simulink library "NonEntVncAppliedBtc"  (R2022b)
settings: Solver=VariableStepAuto  StartTime=0.0  StopTime=10.0  RelTol=1e-3
values from neighbouring files (symbols this model uses):
  den = [b1 b2]    [firstOrderButter.m]
  num = [a1 a2]    [firstOrderButter.m]
undefined symbols (not defined in the file or in its folder): Row
libraries: TuneVar x4, TOP x2, FeaturePath x1, HandyTextFile x1, dspsigops x1, AudioStats x1
settings Model: Creator=kl13806  LastModifiedBy=kl13806
settings SolverCC: AlgebraicLoopSolver=TrustRegion
settings DebuggingCC: UnconnectedInputMsg=warning  UnconnectedOutputMsg=warning  UnconnectedLineMsg=warning  SFMachineParentedDataDiag=warning
settings ModelReferenceCC: EnableRefExpFcnMdlSchedulingChecks=on
settings RTWCC: DLArmComputeVersion=19.05

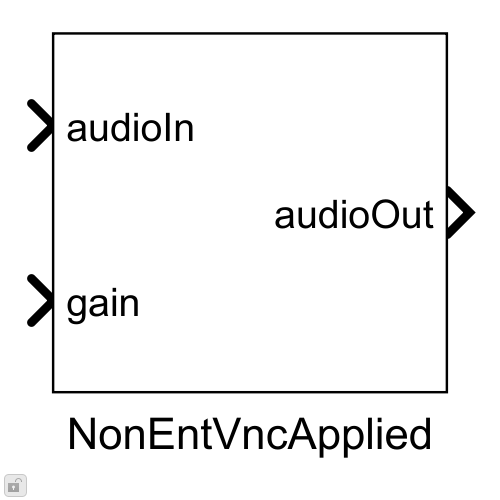
[thumbnail: Simulink's stored preview of the top-level diagram]
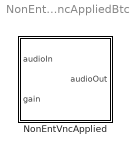
== system NonEntVncAppliedBtc ==
  NonEntVncApplied : Subsystem  mask(Blocklib NonEntVncApplied){Config=[], FeatureName=VNC}
      mask prompts: Config "NonEntVncAppliedConfig"; FeatureName "Feature path name:"
      mask init:
      | blkh=gcbh;
      | Config=BTConfig.Assert(blkh,Config);
      | Config.Validate();
      | BTConfig.InitSetFeatureIfPresent(blkh,'FeatureName');
      mask Callback Config: BTConfig.CallbackHideIfPresent(gcbh,{'FeatureName'});
      mask TypeOptions FeatureName: FeaturePath/FeatureName

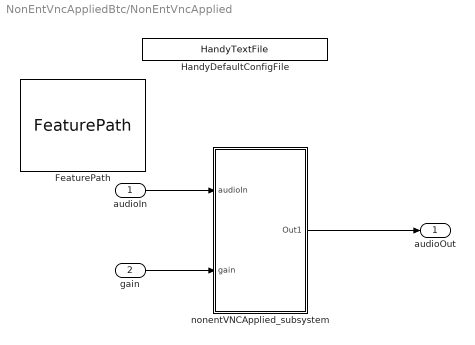
== system NonEntVncAppliedBtc/NonEntVncApplied ==
  audioIn : Inport
  gain : Inport  Port=2
  FeaturePath : FeaturePath/FeaturePath  FeatureName=VNC  IsGroup=off  GroupNumber=-1  IsModule=off  TriggerInit=[500 179 625 271]
      settings: SourceProductName=Bose Talaria
  HandyDefaultConfigFile : HandyTextFile/HandyTextFile  TemplateSource=Config  FileSuffix=Init  OpenDialogOnLoad=off  UseThisBlockName=off  AddGrandParentNamePrefix=off  TheDefaultText=|  ShowInLibBrowser=on
      | % $(FILENAME) Setup model parameters for each "Init" callback (e.g. update diagram)
      | sample_rate_in_hertz = 44100;
      | frame_size = 32;
      | sysin_channel_count = 2;
      settings: SourceProductName=Bose Talaria
  nonentVNCApplied_subsystem : Subsystem
  audioOut : Outport  VectorParamsAs1DForOutWhenUnconnected=off
  wires:
  audioIn/1 -> nonentVNCApplied_subsystem/1(audioIn)
  gain/1 -> nonentVNCApplied_subsystem/2(gain)
  nonentVNCApplied_subsystem/1(Out1) -> audioOut/1

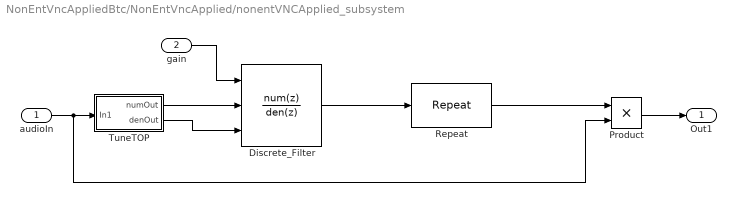
== system NonEntVncAppliedBtc/NonEntVncApplied/nonentVNCApplied_subsystem ==
  audioIn : Inport
  gain : Inport  Port=2
  Discrete_Filter : DiscreteFilter  NumeratorSource=Input port  Numerator=num  DenominatorSource=Input port  Denominator=den  InputProcessing=Columns as channels (frame based)  FilterStructure=Direct form II transposed  a0EqualsOne=on
      settings: InputPortMap=u0,p1,p3
  Product : Product
  Repeat : dspsigops/Repeat  N=Config.FrameSize  InputProcessing=Columns as channels (frame based)  RateOptions=Enforce single-rate processing  ic=0  mode=Unused parameter value
  TuneTOP : Subsystem
  Out1 : Outport  VectorParamsAs1DForOutWhenUnconnected=off
  wires:
  Repeat/1 -> Product/1
  Discrete_Filter/1 -> Repeat/1
  Product/1 -> Out1/1
  gain/1 -> Discrete_Filter/1
  TuneTOP/1(numOut) -> Discrete_Filter/2
  TuneTOP/2(denOut) -> Discrete_Filter/3
  audioIn/1 -> Product/2, TuneTOP/1(In1)

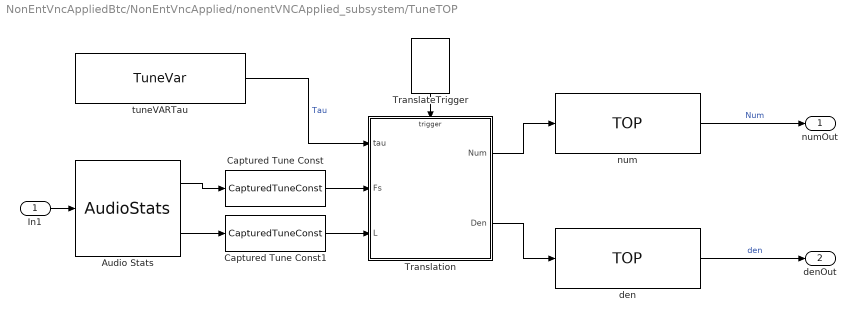
== system NonEntVncAppliedBtc/NonEntVncApplied/nonentVNCApplied_subsystem/TuneTOP ==
  In1 : Inport
  Audio Stats : AudioStats/AudioStats  DoSampleRate=on  TypeSampleRate=Inherit: auto  DoCallRate=off  TypeCallRate=Inherit: auto  DoFrameSize=on  TypeFrameSize=Inherit: auto  DoChannelCount=off  TypeChannelCount=Inherit: auto  DoTaskRateFactor=off  TypeTaskRateFactor=Inherit: auto  MacroNameRoot=AUDIO  MacroNameRootEval='AUDIO'  IsMacroNameEval=off  MacroSampleRate=off  MacroCallRate=off  MacroFrameSize=off  MacroChannelCount=off  MacroTaskRateFactor=off  MacroTaskId=off  ValidateSampleRate=off  ValueSampleRate=[]  ValidateCallRate=off  ValueCallRate=[]  ValidateFrameSize=off  ValueFrameSize=[]  ValidateChannelCount=off  ValueChannelCount=[]  ValidateTaskRateFactor=off  ValueTaskRateFactor=[]
      settings: SourceProductName=Bose Talaria
  Captured Tune Const : TuneVar/CapturedTuneConst  TriggerInit=[120 32 220 68]  Role=Automatic
      settings: SourceProductName=Bose Talaria
  Captured Tune Const1 : TuneVar/CapturedTuneConst  TriggerInit=[120 77 220 113]  Role=Automatic
      settings: SourceProductName=Bose Talaria
  TranslateTrigger : TuneVar/TranslateTrigger  TriggerInit=[306 -100 344 -45]
      settings: SourceProductName=Bose Talaria
  Translation : MATLAB Function  TreatAsAtomicUnit=on
  den : TOP/TOP  TriggerInit=[450 90 595 150]  TopName=den  DataType=single  BankNumber=0  PreOverlay=false  PostOverlay=false  Role=Automatic
      settings: SourceProductName=Bose Talaria
  num : TOP/TOP  TriggerInit=[450 -45 595 15]  TopName=Num  DataType=single  BankNumber=0  PreOverlay=false  PostOverlay=false  Role=Automatic
      settings: SourceProductName=Bose Talaria
  tuneVARTau : TuneVar/TuneVar  TuneName=Tau  SpecifyMaxSize=on  VariableDim=1 (Row)  MaxSize=[1 1]  TunabilityNumber=1  MinValue=[]  MaxValue=[]  TriggerInit=[-30 -85 140 -35]  MaskValue=Config.DefaultTau
      settings: SourceProductName=Bose Talaria
  numOut : Outport  VectorParamsAs1DForOutWhenUnconnected=off
  denOut : Outport  Port=2  VectorParamsAs1DForOutWhenUnconnected=off
  wires:
  In1/1 -> Audio Stats/1
  num/1 -> numOut/1  "Num"
  den/1 -> denOut/1  "den"
  TranslateTrigger/1 -> Translation/Trigger
  tuneVARTau/1 -> Translation/1(tau)  "Tau"
  Audio Stats/1 -> Captured Tune Const/1
  Audio Stats/2 -> Captured Tune Const1/1
  Translation/1(Num) -> num/1
  Translation/2(Den) -> den/1
  Captured Tune Const/1 -> Translation/2(Fs)
  Captured Tune Const1/1 -> Translation/3(L)

== matlab function NonEntVncAppliedBtc/NonEntVncApplied/nonentVNCApplied_subsystem/TuneTOP/Translation ==
  data: Num output; tau input; Fs input; L input; Den output
  events: trigger input FUNCTION_CALL_EVENT
function [Num, Den]  = fcn(tau, Fs, L)

f0 = 1/tau.Value;   % Approximation of cutoff freq from lpf filter time constant

fs_lpf = Fs/L;        % lpf filtter sample rate

% [Num, Den]= butter(1,2*f0/fs_lpf);  % butter() doesn't work with dynamic parameters
[Num, Den] = firstOrderButter(fs_lpf,f0);  % Calculation of lpf filter coefficients
